simulink model "V3_2_MatlabFn"  (R2017b)
settings: Solver=VariableStepAuto  StartTime=0.0  StopTime=.1  MaxStep=1e-4  RelTol=1e-3
undefined symbols (not defined in the file or in its folder): gain, Ion, L, Lithium, RL
libraries: powerlib x55, simulink x11, nesl_utility x5, fl_lib x4, powerlib_meascontrol x4, elec_lib x3, electricdrivelib x2, simulink_need_slupdate x1, dspswit3 x1
settings Model: Creator=Manu Krishnan  LastModifiedBy=Manu Krishnan

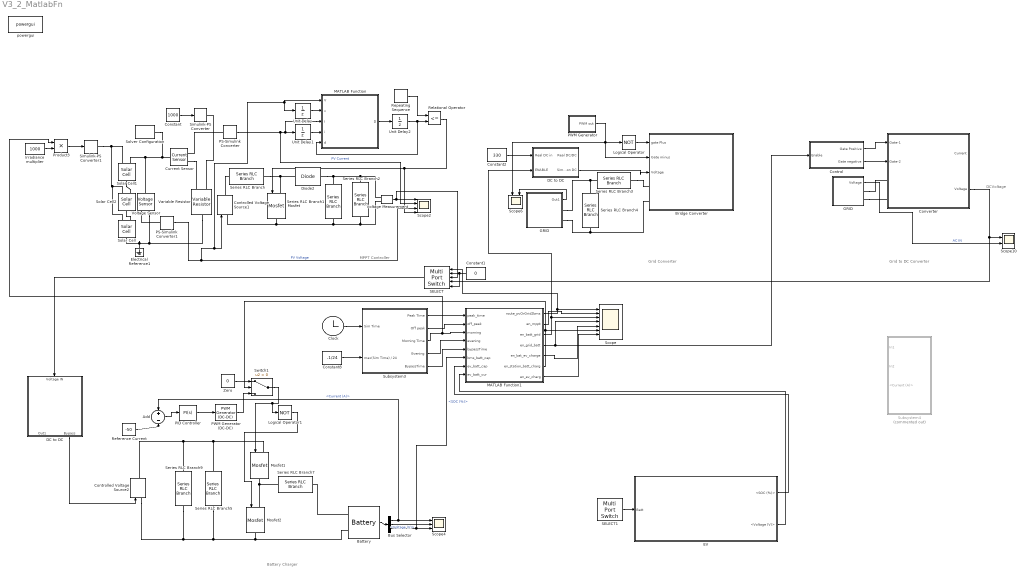
== system V3_2_MatlabFn ==
  note: DCVoltage
  note: Grid Converter
  note: Battery Charger
  note: MPPT Controller
  note: Grid to DC Converter
  Add : Sum  Inputs=+-
  Battery : electricdrivelib/Extra Sources/Battery  BatType=Lithium-Ion  ShowTempParam=off  ThermalPreset=no  ShowAgeParam=on  NomV=300  NomQ=100  SOC=30  Batt_Tr=1  PresetModel=on  MaxQ=100  MinV=225  FullV=349.1961  Dis_rate=43.4783  R=0.03  Normal_OP=90.4348  expZone="[324.1158      4.913043]"  current=[6.5 13 32.5]  Units=Time  Tci=20  NomT=20  T2=-30  MaxQ2=4.8  FullV2=7.1  Normal_OP2=5.655  expZone2="[6.58           1]"  Rca=0.6  ti=2000  Dp=0  Neq0=0  Tsim=1e6  Ta1=25  Qeol=5.4*0.9  Reol=0.013333*1.2  Char_age=[2.3478, 3]  Dis_age=[2.3478, 10]  N1=1500  N2=10500  N3=1000  N4=1400  Ta2=45  N5=950
  Bridge Converter : Subsystem
  Bus Selector : BusSelector  OutputSignals=Current (A),Voltage (V),SOC (%)
  Clock : Clock
  Constant : Constant  Value=1000
  Constant1 : Constant  Value=0
  Constant2 : Constant  Value=330
  Constant8 : Constant  Value=.1/24  VectorParams1D=off
  Control : Subsystem
  Controlled Voltage Source1 : powerlib/Electrical Sources/Controlled Voltage Source  Initialize=on  Source_Type=DC  Amplitude=0  Phase=0  Frequency=0  Measurements=None
  Controlled Voltage Source2 : powerlib/Electrical Sources/Controlled Voltage Source  Initialize=on  Source_Type=DC  Amplitude=0  Phase=0  Frequency=0  Measurements=None
  Converter : Subsystem
  Current Sensor : fl_lib/Electrical/Electrical Sensors/Current Sensor
  DC to DC : Subsystem
  "DC to DC " : Subsystem
  Diode2 : powerlib/Power Electronics/Diode  Ron=0.001  Lon=0  Vf=0.8  IC=0  UseSnubber=0  Rs=500  Cs=250e-9  Measurements=off
  EV : Subsystem
      mask Display: image('C:\Users\Manu Krishnan\Downloads\White-Tesla-Electric-Car-PNG-Free-Download (1).png');
  Electrical Reference1 : fl_lib/Electrical/Electrical Elements/Electrical Reference
  GRID : Subsystem
  "GRID " : Subsystem
  Irradiance multiplier : Constant  Value=1000
  Logical Operator : Logic  Operator=NOT  AllPortsSameDT=off  OutDataTypeStr=boolean
  Logical Operator1 : Logic  Operator=NOT  IconShape=distinctive  AllPortsSameDT=off  OutDataTypeStr=boolean
  MATLAB Function : MATLAB Function  TreatAsAtomicUnit=on
  MATLAB Function1 : MATLAB Function  TreatAsAtomicUnit=on
  Mosfet : powerlib/Power Electronics/Mosfet  Ron=0.1  Lon=0  Rd=0.01  Vfd=0  IC=0  Rs=1e5  Cs=inf  Measurements=off
  Mosfet1 : powerlib/Power Electronics/Mosfet  Ron=0.1  Lon=0  Rd=0.01  Vfd=0  IC=0  Rs=1e5  Cs=inf  Measurements=off
  Mosfet2 : powerlib/Power Electronics/Mosfet  Ron=0.1  Lon=0  Rd=0.01  Vfd=0  IC=0  Rs=1e5  Cs=inf  Measurements=off
  PID Controller : simulink/Continuous/PID Controller  Controller=PI  TimeDomain=Continuous-time  SampleTime=-1  IntegratorMethod=Forward Euler  FilterMethod=Forward Euler  Form=Parallel  UseFilter=on  ControllerParametersSource=internal  P=.005  I=10  D=0  N=100  InitialConditionSource=internal  InitialConditionForIntegrator=0  InitialConditionForFilter=0  ExternalReset=none  LimitOutput=on  UpperSaturationLimit=0.975  LowerSaturationLimit=-inf  LinearizeAsGain=on  AntiWindupMode=none  Kb=1  TrackingMode=off  Kt=1  PParamMin=[]  PParamMax=[]  IParamMin=[]  IParamMax=[]  DParamMin=[]  DParamMax=[]  NParamMin=[]  NParamMax=[]  KbParamMin=[]  KbParamMax=[]  KtParamMin=[]  KtParamMax=[]  POutMin=[]  POutMax=[]  IOutMin=[]  IOutMax=[]  DOutMin=[]  DOutMax=[]  NOutMin=[]  NOutMax=[]  KbOutMin=[]  KbOutMax=[]  KtOutMin=[]  KtOutMax=[]  IntegratorOutMin=[]  IntegratorOutMax=[]  FilterOutMin=[]  FilterOutMax=[]  SumOutMin=[]  SumOutMax=[]  SumI1OutMin=[]  SumI1OutMax=[]  SumI2OutMin=[]  SumI2OutMax=[]  SumI3OutMin=[]  SumI3OutMax=[]  SumDOutMin=[]  SumDOutMax=[]  SaturationOutMin=[]  SaturationOutMax=[]  IntegratorContinuousStateAttributes=''  IntegratorStateMustResolveToSignalObject=off  IntegratorRTWStateStorageClass=Auto  FilterContinuousStateAttributes=''  FilterStateMustResolveToSignalObject=off  FilterRTWStateStorageClass=Auto  DifferentiatorICPrevScaledInput=0  DifferentiatorOutMin=[]  DifferentiatorOutMax=[]  InitialConditionSetting=State (most efficient)  FilterDiffOutCoefMin=[]  FilterDiffOutCoefMax=[]  SumDenOutMin=[]  SumDenOutMax=[]  SumNumOutMin=[]  SumNumOutMax=[]  ReciprocalOutMin=[]  ReciprocalOutMax=[]  DivideOutMin=[]  DivideOutMax=[]  TunerSelectOption=Transfer Function Based (PID Tuner App)
  PS-Simulink Converter : nesl_utility/PS-Simulink Converter  PhysicalDomain=network_engine_domain  SubClassName=ps_output  LeftPortType=input  RightPortType=output  PseudoPeriodic=off  Frequencies=[]  Unit=1  AffineConversion=off
  PS-Simulink Converter1 : nesl_utility/PS-Simulink Converter  PhysicalDomain=network_engine_domain  SubClassName=ps_output  LeftPortType=input  RightPortType=output  PseudoPeriodic=off  Frequencies=[]  Unit=1  AffineConversion=off
  PWM Generator : Subsystem
  PWM Generator (DC-DC) : powerlib_meascontrol/Pulse & Signal Generators/PWM Generator (DC-DC)  Fsw=5000  Ts=5e-6
  Product3 : Product
  Reference Current : Constant  Value=-50
  Relational Operator : RelationalOperator  Operator=<=  OutDataTypeStr=boolean  RndMeth=Simplest
  Repeating Sequence : simulink/Sources/Repeating Sequence  rep_seq_t=[0 0.5 1]/1000  rep_seq_y=[0 1 0]
  SELECT : MultiPortSwitch  DataPortOrder=Zero-based contiguous  DataPortForDefault=Additional data port
  SELECT1 : MultiPortSwitch  DataPortOrder=Zero-based contiguous  DataPortForDefault=Additional data port
  Scope : Scope  NumInputPorts=7
  Scope10 : Scope  NumInputPorts=2
  Scope2 : Scope  NumInputPorts=4
  Scope4 : Scope  NumInputPorts=3
  Scope6 : Scope  NumInputPorts=2
  Series RLC Branch : powerlib/Elements/Series RLC Branch  LConnTagsString=__new0  RConnTagsString=__new0  BranchType=L  Resistance=1  Inductance=1000e-6  SetiL0=off  InitialCurrent=0  Capacitance=1e-6  Setx0=off  InitialVoltage=0  Measurements=None
  Series RLC Branch1 : powerlib/Elements/Series RLC Branch  LConnTagsString=__new0  RConnTagsString=__new0  BranchType=C  Resistance=1  Inductance=100e-3  SetiL0=off  InitialCurrent=0  Capacitance=1000e-6  Setx0=off  InitialVoltage=0  Measurements=None
  Series RLC Branch2 : powerlib/Elements/Series RLC Branch  LConnTagsString=__new0  RConnTagsString=__new0  BranchType=R  Resistance=10  Inductance=100e-3  SetiL0=off  InitialCurrent=0  Capacitance=1e-6  Setx0=off  InitialVoltage=0  Measurements=None
  Series RLC Branch3 : powerlib/Elements/Series RLC Branch  LConnTagsString=__new0  RConnTagsString=__new0  BranchType=L  Resistance=1  Inductance=1e-3  SetiL0=off  InitialCurrent=0  Capacitance=1e-6  Setx0=off  InitialVoltage=0  Measurements=None
  Series RLC Branch4 : powerlib/Elements/Series RLC Branch  LConnTagsString=__new0  RConnTagsString=__new0  BranchType=C  Resistance=1  Inductance=100e-3  SetiL0=off  InitialCurrent=0  Capacitance=100e-6  Setx0=off  InitialVoltage=0  Measurements=None
  Series RLC Branch5 : powerlib/Elements/Series RLC Branch  LConnTagsString=__new0  RConnTagsString=__new0  BranchType=RC  Resistance=0.0001  Inductance=100e-3  SetiL0=off  InitialCurrent=0  Capacitance=1000e-6  Setx0=off  InitialVoltage=0  Measurements=None
  Series RLC Branch7 : powerlib/Elements/Series RLC Branch  LConnTagsString=__new0  RConnTagsString=__new0  BranchType=RL  Resistance=.1  Inductance=5.8e-4  SetiL0=off  InitialCurrent=0  Capacitance=1e-6  Setx0=off  InitialVoltage=0  Measurements=None
  Series RLC Branch9 : powerlib/Elements/Series RLC Branch  LConnTagsString=__new0  RConnTagsString=__new0  BranchType=R  Resistance=100  Inductance=100e-3  SetiL0=off  InitialCurrent=0  Capacitance=1e-6  Setx0=off  InitialVoltage=0  Measurements=None
  Simulink-PS Converter : nesl_utility/Simulink-PS Converter  PhysicalDomain=network_engine_domain  SubClassName=ps_input  LeftPortType=input  RightPortType=output  PseudoPeriodic=off  Frequencies=[]  NoiseDistribution=none  NoiseParameters=[]  Unit=1  AffineConversion=off  FilteringAndDerivatives=provide  SimscapeFilterOrder=1  InputFilterTimeConstant=0.001  UdotUserProvided=0
  Simulink-PS Converter1 : nesl_utility/Simulink-PS Converter  PhysicalDomain=network_engine_domain  SubClassName=ps_input  LeftPortType=input  RightPortType=output  PseudoPeriodic=off  Frequencies=[]  NoiseDistribution=none  NoiseParameters=[]  Unit=1  AffineConversion=off  FilteringAndDerivatives=provide  SimscapeFilterOrder=1  InputFilterTimeConstant=0.001  UdotUserProvided=0
  Solar Cell : elec_lib/Sources/Solar Cell  prm=1  Isc=7.34 A  Voc=3.356 V  Is=1e-6 A  Is2=0 A  Iph=7.34 A  Ir0=1000 W/m^2  ec=1.5  N2=2  Rs=0 Ohm  Rp=inf Ohm  N_series=1  TIPH1=0 1/K  EG=1.11 eV  TXIS1=3  TXIS2=3  TRS1=0  TRP1=0  Tmeas=25 degC  TFIXED=25 degC  thermal_mass=100 J/K  initial_temperature=25 degC
      settings: SourceProductName=Simscape Electronics  SourceProductBaseCode=SN
  Solar Cell1 : elec_lib/Sources/Solar Cell  prm=1  Isc=7.34 A  Voc=3.356 V  Is=1e-6 A  Is2=0 A  Iph=7.34 A  Ir0=1000 W/m^2  ec=1.5  N2=2  Rs=0 Ohm  Rp=inf Ohm  N_series=1  TIPH1=0 1/K  EG=1.11 eV  TXIS1=3  TXIS2=3  TRS1=0  TRP1=0  Tmeas=25 degC  TFIXED=25 degC  thermal_mass=100 J/K  initial_temperature=25 degC
      settings: SourceProductName=Simscape Electronics  SourceProductBaseCode=SN
  Solar Cell2 : elec_lib/Sources/Solar Cell  prm=1  Isc=7.34 A  Voc=3.356 V  Is=1e-6 A  Is2=0 A  Iph=7.34 A  Ir0=1000 W/m^2  ec=1.5  N2=2  Rs=0 Ohm  Rp=inf Ohm  N_series=1  TIPH1=0 1/K  EG=1.11 eV  TXIS1=3  TXIS2=3  TRS1=0  TRP1=0  Tmeas=25 degC  TFIXED=25 degC  thermal_mass=100 J/K  initial_temperature=25 degC
      settings: SourceProductName=Simscape Electronics  SourceProductBaseCode=SN
  Solver Configuration : nesl_utility/Solver Configuration  PhysicalDomain=network_engine_domain  SubClassName=solver  LeftPortType=input  RightPortType=generic  Accelerate=off  Tones=[]  Harmonics=[]  SimulateNoise=off  Profile=off  UseLocalSampling=off  EnableSwitchedLinearOptims=on  FrequencyDomain=off  UseCCode=off  RelTol=0.001  AbsTol=1e-06  MinStep=1e-09  ToWorkspace=off  RevertToSquareIcSolve=off  NumHomotopyIterations=100  PhasorMode=off  PhasorModeNumHarmonics=1  DoDC=off  ResidualTolerance=1e-09  UseLocalSolver=off  LocalSolverChoice=NE_BACKWARD_EULER_ADVANCER  LocalSolverSampleTime=0.001  DoFixedCost=off  MaxNonlinIter=3  MaxModeIter=2  LinearAlgebra=Sparse  DelaysMemoryBudget=1024  AutomaticFiltering=on  FilteringTimeConstant=0.001
  Subsystem3 : Subsystem
  Subsystem4 : Subsystem  Commented=on
  Switch1 : Switch  Criteria=u2 > Threshold
  Unit Delay : UnitDelay  SampleTime=-1
  Unit Delay1 : UnitDelay  SampleTime=-1
  Unit Delay2 : UnitDelay  SampleTime=-1
  Variable Resistor : fl_lib/Electrical/Electrical Elements/Variable Resistor  Rmin=0 Ohm  i_specify=off  i_priority=None  i=0 A  i_nominal_specify=off  i_nominal_unit=A  i_nominal_value=1  v_specify=off  v_priority=None  v=0 V  v_nominal_specify=off  v_nominal_unit=V  v_nominal_value=1
  Voltage Measurement : powerlib/Measurements/Voltage Measurement  PhasorSimulation=off  OutputType=Complex  PSBequivalent=0
  Voltage Sensor : fl_lib/Electrical/Electrical Sensors/Voltage Sensor
  Zero : Constant  Value=0
  powergui : powerlib/powergui  Priority=1  SimulationMode=Continuous  SampleTime=50e-6  frequency=60  Iterations=50  frequencyindice=0  Pbase=100e6  ErrMax=1e-4  UnitsV=kV  UnitsW=MW  buscounter=0  FunctionMessages=off  echomessages=off  EnableUseOfTLC=off  CurrentSourceSwitches=off  DisableSnubberDevices=off  DisableRonSwitches=off  DisableVfSwitches=off  DisplayEquations=off  SolverType=Tustin/Backward Euler (TBE)  Interpol=off  ExternalGateDelay=off  methode=off  Ts=100  x0status=blocks  SPID=on  SwTol=0  HookPort=off  RestoreLinks=warning  ResistiveCurrentMeasurement=off  Frange=[0:2:500]  Ylog=off  Xlog=on  ShowGrid=off  save=off  variable=ZData  structure=0  ZoomFFT=off  StartTime=0.0  cycles=1  DisplayStyle=1  fundamental=60  FreqAxis=off  MaxFrequency=1000  frequencyindicesteady=1  RmsSteady=1  display=off
  wires:
  Constant/1 -> Simulink-PS Converter/1
  PS-Simulink Converter/1 -> Scope2/2, MATLAB Function/3(I), Unit Delay1/1  "PV Current"
  PS-Simulink Converter1/1 -> Unit Delay/1, MATLAB Function/1(V), Controlled Voltage Source1/1, Scope2/3  "PV Voltage"
  Voltage Measurement/1 -> SELECT/3, Scope2/1
  Unit Delay/1 -> MATLAB Function/2(v)
  Unit Delay1/1 -> MATLAB Function/4(i)
  MATLAB Function/1(D) -> Unit Delay2/1
  Unit Delay2/1 -> Relational Operator/2, MATLAB Function/5(d)
  Repeating Sequence/1 -> Relational Operator/1
  Logical Operator/1 -> Bridge Converter/1(gate Plus)
  PWM Generator/1("PWM out ") -> Scope6/1, Bridge Converter/2(Gate minus), Logical Operator/1
  Battery/1 -> Bus Selector/1
  Bus Selector/1 -> Add/1, Scope4/1  "<Current (A)>"
  Bus Selector/3 -> MATLAB Function1/6(bms_batt_cap), Scope4/3  "<SOC (%)>"
  Bus Selector/2 -> Scope4/2  "<Voltage (V)>"
  PID Controller/1 -> PWM Generator (DC-DC)/1
  Logical Operator1/1 -> Mosfet2/1
  Add/1 -> PID Controller/1
  Reference Current/1 -> Add/2
  Control/2(Gate negative) -> Converter/2(Gate-2)
  Control/1(Gate Positive) -> Converter/1(Gate-1)
  "GRID "/1(Voltage) -> Scope10/2  "AC IN"
  Switch1/1 -> Mosfet1/1, Logical Operator1/1
  PWM Generator (DC-DC)/1 -> Switch1/3
  Clock/1 -> Subsystem3/1(Sim Time)
  Constant8/1 -> Subsystem3/2(max(Sim Time) / 24)
  GRID/1(Out1) -> Scope6/2
  Converter/2(Voltage) -> Scope10/1, SELECT/4
  Subsystem3/1(Peak Time) -> MATLAB Function1/1(peak_time)
  Subsystem3/2(Off peak) -> MATLAB Function1/2(off_peak)
  Subsystem3/3(Morning Time) -> MATLAB Function1/3(morning), Product3/1
  Subsystem3/4(Evening) -> MATLAB Function1/4(evening)
  Subsystem3/5(BypassTime) -> MATLAB Function1/5(bypassTime)
  MATLAB Function1/2(en_mppt) -> Scope/2
  MATLAB Function1/3(en_batt_grid) -> Scope/3, DC to DC/2(ENABLE)
  MATLAB Function1/7(en_ev_charg) -> Scope/7
  MATLAB Function1/6(en_station_batt_charg) -> Switch1/2, Scope/6
  Zero/1 -> Switch1/1
  Constant1/1 -> SELECT/5, SELECT/2
  MATLAB Function1/1(route_pvOrGrid2bms) -> SELECT/1, Scope/1
  MATLAB Function1/5(en_bat_ev_charge) -> Scope/5
  Relational Operator/1 -> Scope2/4, Mosfet/1
  Irradiance multiplier/1 -> Product3/2
  Product3/1 -> Simulink-PS Converter1/1
  MATLAB Function1/4(en_grid_batt) -> Scope/4, Control/1(Enable)
  DC to DC/2(Simulation DC) -> Bridge Converter/3(Voltage)
  Constant2/1 -> DC to DC/1(Real DC in)
  "DC to DC "/2(Bypass) -> Controlled Voltage Source2/1
  SELECT/1 -> "DC to DC "/1(Voltage IN)
  EV/1(<SOC (%)>) -> MATLAB Function1/7(ev_batt_cap)
  EV/2(<Voltage (V)>) -> MATLAB Function1/8(ev_batt_cur)
  SELECT1/1 -> EV/1(Batt)
  connections:
  Solar Cell1/RConn1 -- Solar Cell2/LConn2
  Solar Cell2/RConn1 -- Solar Cell/LConn2
  Variable Resistor/RConn1 -- Voltage Sensor/RConn2 -- Electrical Reference1/LConn1 -- Solar Cell/RConn1
  Variable Resistor/LConn1 -- Simulink-PS Converter/RConn1
  Simulink-PS Converter1/RConn1 -- Solar Cell/LConn1 -- Solar Cell2/LConn1 -- Solar Cell1/LConn1
  Solar Cell1/LConn2 -- Voltage Sensor/LConn1 -- Solver Configuration/RConn1 -- Current Sensor/LConn1
  Current Sensor/RConn2 -- Variable Resistor/LConn2
  Current Sensor/RConn1 -- PS-Simulink Converter/LConn1
  Series RLC Branch/RConn1 -- Diode2/LConn1 -- Mosfet/LConn1
  Mosfet/RConn1 -- Voltage Measurement/LConn2 -- Series RLC Branch2/RConn1 -- Series RLC Branch1/RConn1 -- Controlled Voltage Source1/LConn1
  Diode2/RConn1 -- Voltage Measurement/LConn1 -- Series RLC Branch2/LConn1 -- Series RLC Branch1/LConn1
  Controlled Voltage Source1/RConn1 -- Series RLC Branch/LConn1
  Series RLC Branch3/LConn1 -- GRID/RConn1 -- Series RLC Branch4/LConn1
  Series RLC Branch3/RConn1 -- Bridge Converter/LConn1
  Series RLC Branch4/RConn1 -- GRID/RConn2 -- Bridge Converter/LConn2
  Mosfet1/RConn1 -- Mosfet2/LConn1 -- Series RLC Branch7/RConn1
  Battery/LConn1 -- Series RLC Branch7/LConn1
  Battery/LConn2 -- Series RLC Branch5/RConn1 -- Controlled Voltage Source2/LConn1 -- Series RLC Branch9/RConn1 -- Mosfet2/RConn1
  Series RLC Branch5/LConn1 -- Controlled Voltage Source2/RConn1 -- Series RLC Branch9/LConn1 -- Mosfet1/LConn1
  "GRID "/RConn1 -- Converter/LConn1
  "GRID "/RConn2 -- Converter/LConn2
  PS-Simulink Converter1/LConn1 -- Voltage Sensor/RConn1

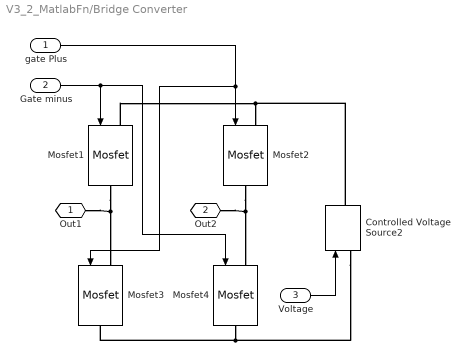
== system V3_2_MatlabFn/Bridge Converter ==
  gate Plus : Inport
  Gate minus : Inport  Port=2
  Voltage : Inport  Port=3
  Controlled Voltage Source2 : powerlib/Electrical Sources/Controlled Voltage Source  Initialize=on  Source_Type=DC  Amplitude=0  Phase=0  Frequency=0  Measurements=None
  Mosfet{1..4} (4 alike) : powerlib/Power Electronics/Mosfet  Ron=0.1  Lon=0  Rd=0.01  Vfd=0  IC=0  Rs=1e5  Cs=inf  Measurements=off
  Out1 : PMIOPort  Port=1  Side=Left
  Out2 : PMIOPort  Port=2  Side=Left
  wires:
  Voltage/1 -> Controlled Voltage Source2/1
  gate Plus/1 -> Mosfet3/1, Mosfet2/1
  Gate minus/1 -> Mosfet4/1, Mosfet1/1
  connections:
  Mosfet1/LConn1 -- Controlled Voltage Source2/RConn1 -- Mosfet2/LConn1
  Mosfet4/RConn1 -- Controlled Voltage Source2/LConn1 -- Mosfet3/RConn1
  Mosfet1/RConn1 -- Out1/RConn1 -- Mosfet3/LConn1
  Mosfet2/RConn1 -- Out2/RConn1 -- Mosfet4/LConn1

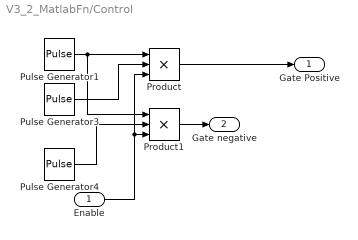
== system V3_2_MatlabFn/Control ==
  Enable : Inport
  Product : Product  Inputs=3
  Product1 : Product  Inputs=3
  Pulse Generator1 : DiscretePulseGenerator  PulseType=Time based  Period=1/25000  PulseWidth=50
  Pulse Generator3 : DiscretePulseGenerator  PulseType=Time based  Period=0.02  PulseWidth=50
  Pulse Generator4 : DiscretePulseGenerator  PulseType=Time based  Period=0.02  PulseWidth=50  PhaseDelay=0.01
  Gate Positive : Outport
  Gate negative : Outport  Port=2
  wires:
  Pulse Generator3/1 -> Product/2
  Pulse Generator1/1 -> Product/1, Product1/1
  Product/1 -> Gate Positive/1
  Product1/1 -> Gate negative/1
  Pulse Generator4/1 -> Product1/2
  Enable/1 -> Product1/3, Product/3

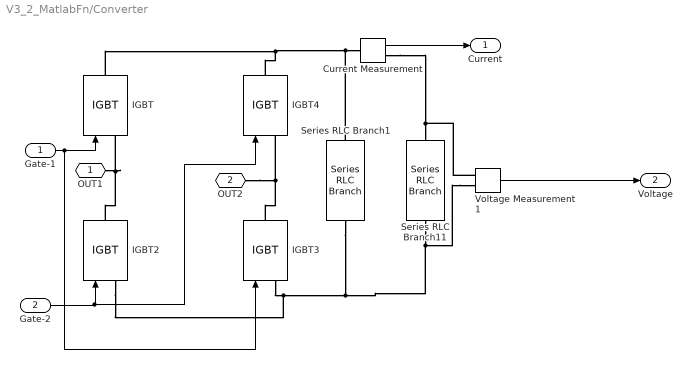
== system V3_2_MatlabFn/Converter ==
  Gate-1 : Inport
  Gate-2 : Inport  Port=2
  Current Measurement : powerlib/Measurements/Current Measurement  PhasorSimulation=off  OutputType=Complex  PSBequivalent=0
  IGBT{,2..4} (4 alike) : powerlib/Power Electronics/IGBT  Ron=0.001  Lon=0  Vf=1  Tf=1e-6  Tt=2e-6  IC=0  Rs=1e5  Cs=inf  Measurements=off
  Series RLC Branch1 : powerlib/Elements/Series RLC Branch  LConnTagsString=__new0  RConnTagsString=__new0  BranchType=C  Resistance=1  Inductance=1e-3  SetiL0=off  InitialCurrent=0  Capacitance=1000e-6  Setx0=off  InitialVoltage=0  Measurements=None
  Series RLC Branch11 : powerlib/Elements/Series RLC Branch  LConnTagsString=__new0  RConnTagsString=__new0  BranchType=R  Resistance=1000  Inductance=1e-3  SetiL0=off  InitialCurrent=0  Capacitance=1e-6  Setx0=off  InitialVoltage=0  Measurements=None
  Voltage Measurement1 : powerlib/Measurements/Voltage Measurement  PhasorSimulation=off  OutputType=Complex  PSBequivalent=0
  OUT1 : PMIOPort  Port=1  Side=Left
  OUT2 : PMIOPort  Port=2  Side=Left
  Current : Outport
  Voltage : Outport  Port=2
  wires:
  Voltage Measurement1/1 -> Voltage/1
  Gate-1/1 -> IGBT3/1, IGBT/1
  Gate-2/1 -> IGBT4/1, IGBT2/1
  Current Measurement/1 -> Current/1
  connections:
  Voltage Measurement1/LConn2 -- Series RLC Branch1/RConn1 -- IGBT2/LConn1 -- IGBT3/LConn1 -- Series RLC Branch11/RConn1
  IGBT4/RConn1 -- IGBT/RConn1 -- Series RLC Branch1/LConn1 -- Current Measurement/LConn1
  Series RLC Branch11/LConn1 -- Current Measurement/RConn1 -- Voltage Measurement1/LConn1
  IGBT/LConn1 -- IGBT2/RConn1 -- OUT1/RConn1
  IGBT4/LConn1 -- IGBT3/RConn1 -- OUT2/RConn1

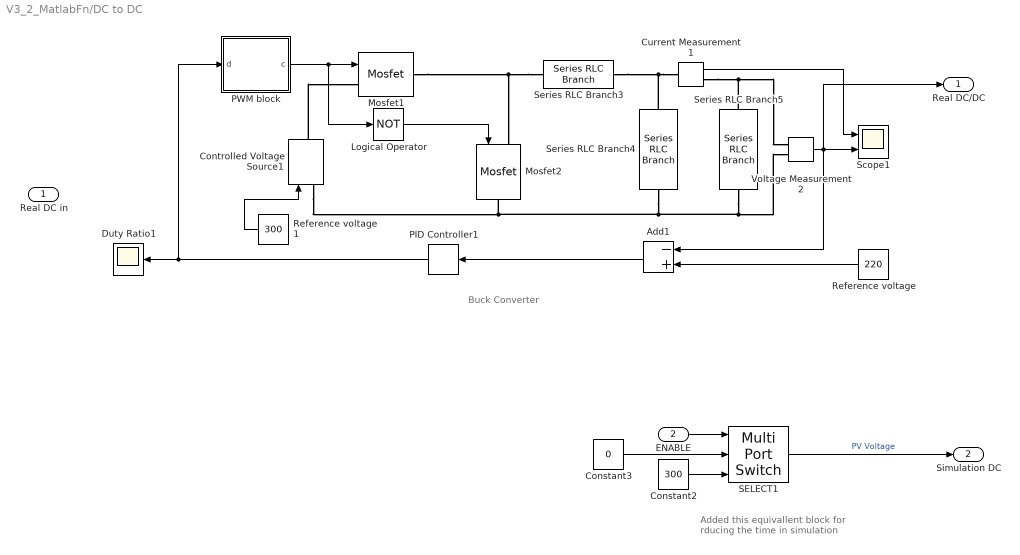
== system V3_2_MatlabFn/DC to DC ==
  note: Added this equivallent block for
      | rducing the time in simulation
  note: Buck Converter
  Real DC in : Inport
  ENABLE : Inport  Port=2
  Add1 : Sum  Inputs=-+
  Constant2 : Constant  Value=300
  Constant3 : Constant  Value=0
  Controlled Voltage Source1 : powerlib/Electrical Sources/Controlled Voltage Source  Initialize=on  Source_Type=DC  Amplitude=200  Phase=0  Frequency=0  Measurements=None
  Current Measurement1 : powerlib/Measurements/Current Measurement  PhasorSimulation=off  OutputType=Complex  PSBequivalent=0
  Duty Ratio1 : Scope
  Logical Operator : Logic  Operator=NOT  AllPortsSameDT=off  OutDataTypeStr=boolean
  Mosfet1 : powerlib/Power Electronics/Mosfet  Ron=0.1  Lon=0  Rd=0.01  Vfd=0  IC=0  Rs=1e5  Cs=inf  Measurements=off
  Mosfet2 : powerlib/Power Electronics/Mosfet  Ron=0.1  Lon=0  Rd=0.01  Vfd=0  IC=0  Rs=1e5  Cs=inf  Measurements=off
  PID Controller1 : simulink_need_slupdate/PID Controller  P=0  I=gain  D=0
      settings: SourceProductName=Simulink
  "PWM block " : Subsystem  mask{fs=100e3}
      mask prompts: fs "Switching fFrequency"
  "Reference voltage   " : Constant  Value=220
  Reference voltage   1 : Constant  Value=300
  SELECT1 : MultiPortSwitch  DataPortOrder=Zero-based contiguous  Inputs=2
  Scope1 : Scope  NumInputPorts=2
  Series RLC Branch3 : powerlib/Elements/Series RLC Branch  LConnTagsString=__new0  RConnTagsString=__new0  BranchType=RL  Resistance=RL  Inductance=L  SetiL0=off  InitialCurrent=0  Capacitance=1e-6  Setx0=off  InitialVoltage=0  Measurements=None
  Series RLC Branch4 : powerlib/Elements/Series RLC Branch  LConnTagsString=__new0  RConnTagsString=__new0  BranchType=R  Resistance=1  Inductance=1e-3  SetiL0=off  InitialCurrent=0  Capacitance=1e-6  Setx0=off  InitialVoltage=0  Measurements=None
  Series RLC Branch5 : powerlib/Elements/Series RLC Branch  LConnTagsString=__new0  RConnTagsString=__new0  BranchType=R  Resistance=1  Inductance=1e-3  SetiL0=off  InitialCurrent=0  Capacitance=1e-6  Setx0=off  InitialVoltage=0  Measurements=None
  Voltage Measurement2 : powerlib/Measurements/Voltage Measurement  PhasorSimulation=off  OutputType=Complex  PSBequivalent=0
  Real DC/DC : Outport
  Simulation DC : Outport  Port=2
  wires:
  PID Controller1/1 -> "PWM block "/1(d), Duty Ratio1/1
  Add1/1 -> PID Controller1/1
  Current Measurement1/1 -> Scope1/1
  "Reference voltage   "/1 -> Add1/2
  "PWM block "/1(c) -> Mosfet1/1, Logical Operator/1
  Logical Operator/1 -> Mosfet2/1
  Voltage Measurement2/1 -> Real DC/DC/1, Scope1/2, Add1/1
  SELECT1/1 -> Simulation DC/1  "PV Voltage"
  Constant3/1 -> SELECT1/2
  ENABLE/1 -> SELECT1/1
  Constant2/1 -> SELECT1/3
  Reference voltage   1/1 -> Controlled Voltage Source1/1
  connections:
  Current Measurement1/LConn1 -- Series RLC Branch4/LConn1 -- Series RLC Branch3/RConn1
  Voltage Measurement2/LConn2 -- Series RLC Branch4/RConn1 -- Controlled Voltage Source1/LConn1 -- Mosfet2/RConn1 -- Series RLC Branch5/RConn1
  Series RLC Branch3/LConn1 -- Mosfet2/LConn1 -- Mosfet1/RConn1
  Current Measurement1/RConn1 -- Series RLC Branch5/LConn1 -- Voltage Measurement2/LConn1
  Controlled Voltage Source1/RConn1 -- Mosfet1/LConn1

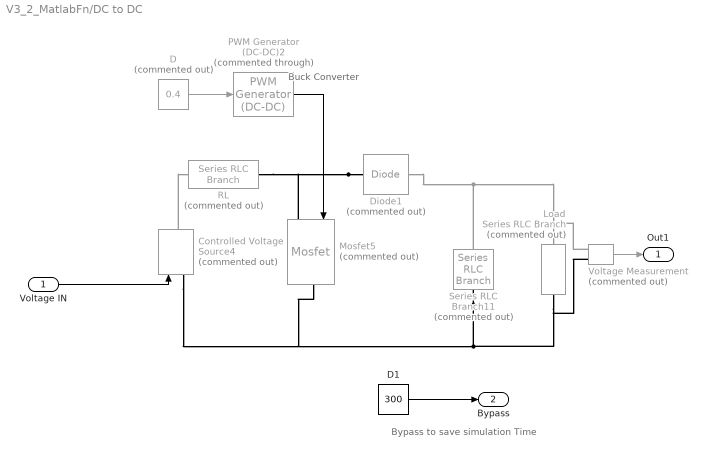
== system V3_2_MatlabFn/DC to DC  ==
  note: Bypass to save simulation Time
  note: Buck Converter
  Voltage IN : Inport
  Controlled Voltage Source4 : powerlib/Electrical Sources/Controlled Voltage Source  Commented=on  Initialize=on  Source_Type=DC  Amplitude=0  Phase=0  Frequency=0  Measurements=None
  D : Constant  Commented=on  Value=0.4
  D1 : Constant  Value=300
  Diode1 : powerlib/Power Electronics/Diode  Commented=on  Ron=1e-3  Lon=0  Vf=0  IC=0  UseSnubber=off  Rs=inf  Cs=inf  Measurements=off
  Load : powerlib/Elements/Series RLC Branch  Commented=on  LConnTagsString=__new0  RConnTagsString=__new0  BranchType=R  Resistance=3  Inductance=200e-6  SetiL0=off  InitialCurrent=0  Capacitance=400e-6  Setx0=off  InitialVoltage=0  Measurements=None
  Mosfet5 : powerlib/Power Electronics/Mosfet  Commented=on  Ron=1e-3  Lon=0  Rd=1e-3  Vfd=0  IC=0  Rs=inf  Cs=inf  Measurements=off
  PWM Generator (DC-DC)2 : powerlib_meascontrol/Pulse & Signal Generators/PWM Generator (DC-DC)  Commented=through  Fsw=20e3  Ts=0
  RL : powerlib/Elements/Series RLC Branch  Commented=on  LConnTagsString=__new0  RConnTagsString=__new0  BranchType=RL  Resistance=1e-3  Inductance=250e-6  SetiL0=off  InitialCurrent=0  Capacitance=1e-6  Setx0=off  InitialVoltage=0  Measurements=None
  Series RLC Branch11 : powerlib/Elements/Series RLC Branch  Commented=on  LConnTagsString=__new0  RConnTagsString=__new0  BranchType=C  Resistance=1e-4  Inductance=200e-6  SetiL0=off  InitialCurrent=0  Capacitance=200e-6  Setx0=off  InitialVoltage=40  Measurements=None
  Voltage Measurement : powerlib/Measurements/Voltage Measurement  Commented=on  PhasorSimulation=off  OutputType=Complex  PSBequivalent=0
  Out1 : Outport
  Bypass : Outport  Port=2
  wires:
  Voltage IN/1 -> Controlled Voltage Source4/1
  D/1 -> PWM Generator (DC-DC)2/1
  PWM Generator (DC-DC)2/1 -> Mosfet5/1
  Voltage Measurement/1 -> Out1/1
  D1/1 -> Bypass/1
  connections:
  Diode1/RConn1 -- Series RLC Branch11/LConn1 -- Voltage Measurement/LConn1 -- Load/LConn1
  Series RLC Branch11/RConn1 -- Voltage Measurement/LConn2 -- Load/RConn1 -- Controlled Voltage Source4/LConn1 -- Mosfet5/RConn1
  Diode1/LConn1 -- RL/RConn1 -- Mosfet5/LConn1
  Controlled Voltage Source4/RConn1 -- RL/LConn1

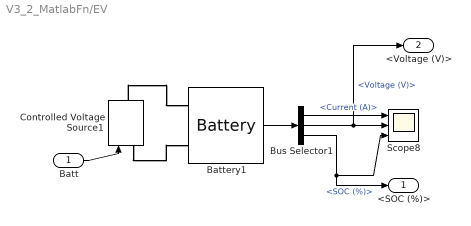
== system V3_2_MatlabFn/EV ==
  Batt : Inport
  Battery1 : electricdrivelib/Extra Sources/Battery  BatType=Lithium-Ion  ShowTempParam=off  ThermalPreset=no  ShowAgeParam=on  NomV=300  NomQ=5.4  SOC=96  Batt_Tr=3  PresetModel=on  MaxQ=5.4  MinV=225  FullV=349.1961  Dis_rate=2.3478  R=0.55556  Normal_OP=4.8835  expZone="[324.1158     0.2653043]"  current=[6.5 13 32.5]  Units=Time  Tci=20  NomT=20  T2=-30  MaxQ2=4.8  FullV2=7.1  Normal_OP2=5.655  expZone2="[6.58           1]"  Rca=0.6  ti=2000  Dp=0  Neq0=0  Tsim=1e6  Ta1=25  Qeol=5.4*0.9  Reol=0.013333*1.2  Char_age=[2.3478, 3]  Dis_age=[2.3478, 10]  N1=1500  N2=10500  N3=1000  N4=1400  Ta2=45  N5=950
  Bus Selector1 : BusSelector  OutputSignals=Current (A),Voltage (V),SOC (%)
  Controlled Voltage Source1 : powerlib/Electrical Sources/Controlled Voltage Source  Initialize=on  Source_Type=DC  Amplitude=0  Phase=0  Frequency=0  Measurements=None
  Scope8 : Scope  NumInputPorts=3
  <SOC (%)> : Outport
  <Voltage (V)> : Outport  Port=2
  wires:
  Bus Selector1/2 -> <Voltage (V)>/1, Scope8/2  "<Voltage (V)>"
  Battery1/1 -> Bus Selector1/1
  Bus Selector1/1 -> Scope8/1  "<Current (A)>"
  Bus Selector1/3 -> <SOC (%)>/1, Scope8/3  "<SOC (%)>"
  Batt/1 -> Controlled Voltage Source1/1
  connections:
  Controlled Voltage Source1/LConn1 -- Battery1/LConn2
  Controlled Voltage Source1/RConn1 -- Battery1/LConn1

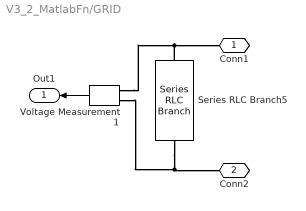
== system V3_2_MatlabFn/GRID ==
  Series RLC Branch5 : powerlib/Elements/Series RLC Branch  LConnTagsString=__new0  RConnTagsString=__new0  BranchType=R  Resistance=1000  Inductance=100e-3  SetiL0=off  InitialCurrent=0  Capacitance=1e-6  Setx0=off  InitialVoltage=0  Measurements=None
  Voltage Measurement1 : powerlib/Measurements/Voltage Measurement  PhasorSimulation=off  OutputType=Complex  PSBequivalent=0
  Conn1 : PMIOPort  Port=1  Side=Right
  Conn2 : PMIOPort  Port=2  Side=Right
  Out1 : Outport
  wires:
  Voltage Measurement1/1 -> Out1/1
  connections:
  Series RLC Branch5/LConn1 -- Conn1/RConn1 -- Voltage Measurement1/LConn2
  Voltage Measurement1/LConn1 -- Conn2/RConn1 -- Series RLC Branch5/RConn1

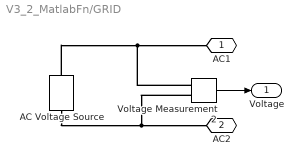
== system V3_2_MatlabFn/GRID  ==
  AC Voltage Source : powerlib/Electrical Sources/AC Voltage Source  Amplitude=230  Phase=0  Frequency=50  SampleTime=0  Measurements=None  BusType=swing  Pref=10e3  Qref=0  Qmin=-inf  Qmax=+inf
  Voltage Measurement2 : powerlib/Measurements/Voltage Measurement  PhasorSimulation=off  OutputType=Complex  PSBequivalent=0
  AC1 : PMIOPort  Port=1  Side=Right
  AC2 : PMIOPort  Port=2  Side=Right
  Voltage : Outport
  wires:
  Voltage Measurement2/1 -> Voltage/1
  connections:
  AC Voltage Source/LConn1 -- AC2/RConn1 -- Voltage Measurement2/LConn2
  AC Voltage Source/RConn1 -- Voltage Measurement2/LConn1 -- AC1/RConn1

== system V3_2_MatlabFn/PWM Generator ==
  Relational Operator1 : RelationalOperator  OutDataTypeStr=boolean  RndMeth=Simplest
  Sawtooth Generator : powerlib_meascontrol/Pulse & Signal Generators/Sawtooth Generator  Freq=10e3  Phase=180  Ts=0
      settings: SourceProductName=Simscape Power Systems
  Sine Wave : Sin  Frequency=314.18  SampleTime=0
  "PWM out " : Outport
  wires:
  Sine Wave/1 -> Relational Operator1/1
  Sawtooth Generator/1 -> Relational Operator1/2
  Relational Operator1/1 -> "PWM out "/1

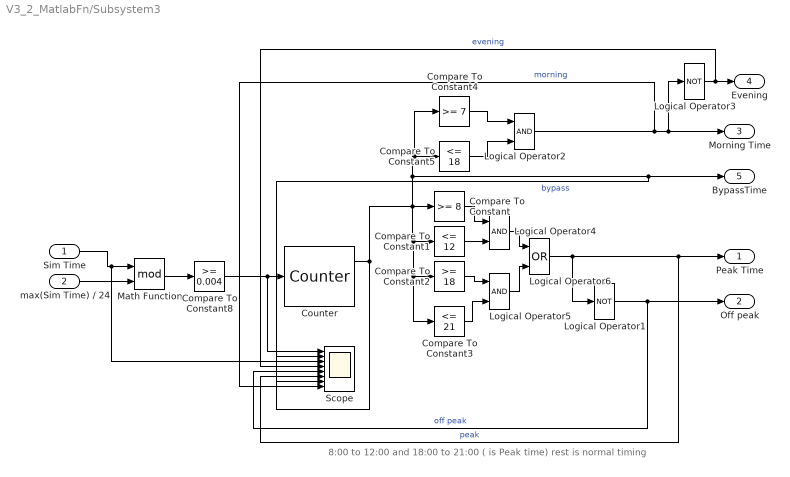
== system V3_2_MatlabFn/Subsystem3 ==
  note: 8:00 to 12:00 and 18:00 to 21:00 ( is Peak time)
      | rest is normal timing
  Sim Time : Inport
  max(Sim Time) / 24 : Inport  Port=2
  Compare To Constant : simulink/Logic and Bit Operations/Compare To Constant  relop=>=  const=8  OutDataTypeStr=boolean  ZeroCross=off
  Compare To Constant1 : simulink/Logic and Bit Operations/Compare To Constant  relop=<=  const=12  OutDataTypeStr=boolean  ZeroCross=off
  Compare To Constant2 : simulink/Logic and Bit Operations/Compare To Constant  relop=>=  const=18  OutDataTypeStr=boolean  ZeroCross=off
  Compare To Constant3 : simulink/Logic and Bit Operations/Compare To Constant  relop=<=  const=21  OutDataTypeStr=boolean  ZeroCross=off
  Compare To Constant4 : simulink/Logic and Bit Operations/Compare To Constant  relop=>=  const=7  OutDataTypeStr=boolean  ZeroCross=off
  Compare To Constant5 : simulink/Logic and Bit Operations/Compare To Constant  relop=<=  const=18  OutDataTypeStr=boolean  ZeroCross=off
  Compare To Constant8 : simulink/Logic and Bit Operations/Compare To Constant  relop=>=  const=0.004  OutDataTypeStr=boolean  ZeroCross=off
  Counter : dspswit3/Counter  Direction=Up  CountEvent=Falling edge  CounterSize=User defined  MaxCount=24  InitialCount=0  Output=Count and Hit  HitValue=24  ResetInput=off  SamplesPerFrame=1  Ts=1  CntDtype=int8  HitDtype=Logical
  Logical Operator1 : Logic  Operator=NOT  AllPortsSameDT=off  OutDataTypeStr=boolean
  Logical Operator2 : Logic  AllPortsSameDT=off  OutDataTypeStr=boolean
  Logical Operator3 : Logic  Operator=NOT  AllPortsSameDT=off  OutDataTypeStr=boolean
  Logical Operator4 : Logic  AllPortsSameDT=off  OutDataTypeStr=boolean
  Logical Operator5 : Logic  AllPortsSameDT=off  OutDataTypeStr=boolean
  Logical Operator6 : Logic  Operator=OR  AllPortsSameDT=off  OutDataTypeStr=boolean
  Math Function : Math  Operator=mod  SaturateOnIntegerOverflow=on
  Scope : Scope  NumInputPorts=8
  Peak Time : Outport
  Off peak : Outport  Port=2
  Morning Time : Outport  Port=3
  Evening : Outport  Port=4
  BypassTime : Outport  Port=5
  wires:
  Sim Time/1 -> Scope/3, Math Function/1
  Logical Operator5/1 -> Logical Operator6/2
  Logical Operator4/1 -> Logical Operator6/1
  Compare To Constant1/1 -> Logical Operator4/2
  Compare To Constant3/1 -> Logical Operator5/2
  Compare To Constant/1 -> Logical Operator4/1
  Logical Operator6/1 -> Logical Operator1/1, Scope/6, Peak Time/1  "peak"
  Math Function/1 -> Compare To Constant8/1
  Logical Operator1/1 -> Scope/5, Off peak/1  "off peak"
  Compare To Constant4/1 -> Logical Operator2/1
  Compare To Constant5/1 -> Logical Operator2/2
  Logical Operator2/1 -> Scope/8, Logical Operator3/1, Morning Time/1  "morning"
  Compare To Constant2/1 -> Logical Operator5/1
  Logical Operator3/1 -> Scope/4, Evening/1  "evening"
  max(Sim Time) / 24/1 -> Math Function/2
  Compare To Constant8/1 -> Scope/1, Counter/1
  Counter/1 -> Scope/2, Scope/7, BypassTime/1, Compare To Constant5/1, Compare To Constant4/1, Compare To Constant3/1, Compare To Constant2/1, Compare To Constant1/1, Compare To Constant/1  "bypass"

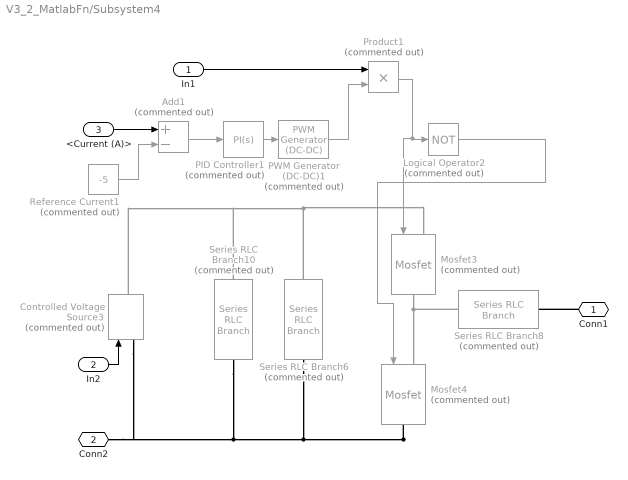
== system V3_2_MatlabFn/Subsystem4 ==
  In1 : Inport
  In2 : Inport  Port=2
  <Current (A)> : Inport  Port=3
  Add1 : Sum  Commented=on  Inputs=+-
  Controlled Voltage Source3 : powerlib/Electrical Sources/Controlled Voltage Source  Commented=on  Initialize=on  Source_Type=DC  Amplitude=0  Phase=0  Frequency=0  Measurements=None
  Logical Operator2 : Logic  Commented=on  Operator=NOT  AllPortsSameDT=off  OutDataTypeStr=boolean
  Mosfet3 : powerlib/Power Electronics/Mosfet  Commented=on  Ron=0.1  Lon=0  Rd=0.01  Vfd=0  IC=0  Rs=1e5  Cs=inf  Measurements=off
  Mosfet4 : powerlib/Power Electronics/Mosfet  Commented=on  Ron=0.1  Lon=0  Rd=0.01  Vfd=0  IC=0  Rs=1e5  Cs=inf  Measurements=off
  PID Controller1 : simulink/Continuous/PID Controller  Commented=on  Controller=PI  TimeDomain=Continuous-time  SampleTime=-1  IntegratorMethod=Forward Euler  FilterMethod=Forward Euler  Form=Parallel  UseFilter=on  ControllerParametersSource=internal  P=.005  I=10  D=0.05  N=100  InitialConditionSource=internal  InitialConditionForIntegrator=0  InitialConditionForFilter=0  ExternalReset=none  LimitOutput=on  UpperSaturationLimit=0.975  LowerSaturationLimit=-inf  LinearizeAsGain=on  AntiWindupMode=none  Kb=1  TrackingMode=off  Kt=1  PParamMin=[]  PParamMax=[]  IParamMin=[]  IParamMax=[]  DParamMin=[]  DParamMax=[]  NParamMin=[]  NParamMax=[]  KbParamMin=[]  KbParamMax=[]  KtParamMin=[]  KtParamMax=[]  POutMin=[]  POutMax=[]  IOutMin=[]  IOutMax=[]  DOutMin=[]  DOutMax=[]  NOutMin=[]  NOutMax=[]  KbOutMin=[]  KbOutMax=[]  KtOutMin=[]  KtOutMax=[]  IntegratorOutMin=[]  IntegratorOutMax=[]  FilterOutMin=[]  FilterOutMax=[]  SumOutMin=[]  SumOutMax=[]  SumI1OutMin=[]  SumI1OutMax=[]  SumI2OutMin=[]  SumI2OutMax=[]  SumI3OutMin=[]  SumI3OutMax=[]  SumDOutMin=[]  SumDOutMax=[]  SaturationOutMin=[]  SaturationOutMax=[]  IntegratorContinuousStateAttributes=''  IntegratorStateMustResolveToSignalObject=off  IntegratorRTWStateStorageClass=Auto  FilterContinuousStateAttributes=''  FilterStateMustResolveToSignalObject=off  FilterRTWStateStorageClass=Auto  DifferentiatorICPrevScaledInput=0  DifferentiatorOutMin=[]  DifferentiatorOutMax=[]  InitialConditionSetting=State (most efficient)  FilterDiffOutCoefMin=[]  FilterDiffOutCoefMax=[]  SumDenOutMin=[]  SumDenOutMax=[]  SumNumOutMin=[]  SumNumOutMax=[]  ReciprocalOutMin=[]  ReciprocalOutMax=[]  DivideOutMin=[]  DivideOutMax=[]  TunerSelectOption=Transfer Function Based (PID Tuner App)
  PWM Generator (DC-DC)1 : powerlib_meascontrol/Pulse & Signal Generators/PWM Generator (DC-DC)  Commented=on  Fsw=5000  Ts=5e-6
  Product1 : Product  Commented=on
  Reference Current1 : Constant  Commented=on  Value=-5
  Series RLC Branch10 : powerlib/Elements/Series RLC Branch  Commented=on  LConnTagsString=__new0  RConnTagsString=__new0  BranchType=R  Resistance=100  Inductance=100e-3  SetiL0=off  InitialCurrent=0  Capacitance=1e-6  Setx0=off  InitialVoltage=0  Measurements=None
  Series RLC Branch6 : powerlib/Elements/Series RLC Branch  Commented=on  LConnTagsString=__new0  RConnTagsString=__new0  BranchType=RC  Resistance=0.0001  Inductance=100e-3  SetiL0=off  InitialCurrent=0  Capacitance=1000e-6  Setx0=off  InitialVoltage=0  Measurements=None
  Series RLC Branch8 : powerlib/Elements/Series RLC Branch  Commented=on  LConnTagsString=__new0  RConnTagsString=__new0  BranchType=RL  Resistance=.1  Inductance=5.8e-4  SetiL0=off  InitialCurrent=0  Capacitance=1e-6  Setx0=off  InitialVoltage=0  Measurements=None
  Conn1 : PMIOPort  Port=1  Side=Left
  Conn2 : PMIOPort  Port=2  Side=Right
  wires:
  <Current (A)>/1 -> Add1/1
  In1/1 -> Product1/1
  PID Controller1/1 -> PWM Generator (DC-DC)1/1
  Logical Operator2/1 -> Mosfet4/1
  PWM Generator (DC-DC)1/1 -> Product1/2
  Product1/1 -> Mosfet3/1, Logical Operator2/1
  Add1/1 -> PID Controller1/1
  Reference Current1/1 -> Add1/2
  In2/1 -> Controlled Voltage Source3/1
  connections:
  Conn1/RConn1 -- Series RLC Branch8/LConn1
  Mosfet3/RConn1 -- Mosfet4/LConn1 -- Series RLC Branch8/RConn1
  Series RLC Branch6/LConn1 -- Controlled Voltage Source3/RConn1 -- Series RLC Branch10/LConn1 -- Mosfet3/LConn1
  Mosfet4/RConn1 -- Series RLC Branch6/RConn1 -- Series RLC Branch10/RConn1 -- Controlled Voltage Source3/LConn1 -- Conn2/RConn1

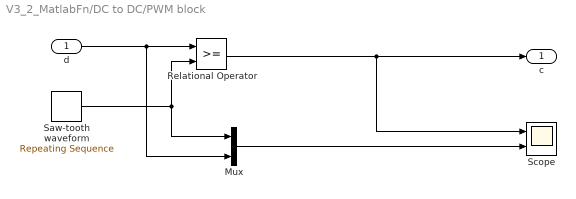
== system V3_2_MatlabFn/DC to DC/PWM block  ==
  d : Inport
  Mux : Mux  Inputs=2
  Relational Operator : RelationalOperator  OutDataTypeStr=boolean  RndMeth=Nearest
  Saw-tooth waveform : simulink/Sources/Repeating Sequence  rep_seq_t=[0 1/fs]  rep_seq_y=[0 1]
  Scope : Scope  NumInputPorts=2
  c : Outport
  wires:
  Mux/1 -> Scope/2
  Relational Operator/1 -> Scope/1, c/1
  Saw-tooth waveform/1 -> Relational Operator/2, Mux/1
  d/1 -> Relational Operator/1, Mux/2

== matlab function V3_2_MatlabFn/MATLAB Function1 ==
  data: route_pvOrGrid2bms output; en_mppt output; en_batt_grid output; en_grid_batt output; en_bat_ev_charge output; en_station_batt_charg output; en_ev_charg output; peak_time input; off_peak input; morning input; evening input; bypassTime input; bms_batt_cap input; ev_batt_cap input; ev_batt_cur input
function [route_pvOrGrid2bms, en_mppt,en_batt_grid, en_grid_batt, en_bat_ev_charge, en_station_batt_charg,en_ev_charg]= Automate(peak_time,off_peak,morning,evening,bypassTime,bms_batt_cap,ev_batt_cap,ev_batt_cur)
from_grid = 2;
from_solar =1;
if(ev_batt_cur < 1)
    carPresent = 0;
else
    carPresent =1;
end

% MODE 1 
% PV to battery
%---------------------------------------------------------------------------------------
%Time	        |Speicific Time	|EV 	             |BatteryBank Capacity	|EV battery
%---------------------------------------------------------------------------------------
%Morning 	    |Off peak	    |Not present         |<80%	                |>90%
%---------------------------------------------------------------------------------------
if  (off_peak &&   carPresent==0 && bms_batt_cap < 80 && ev_batt_cap > 90)
    en_station_batt_charg =1;
    en_mppt =1;
    route_pvOrGrid2bms =from_solar;
    en_batt_grid =0;
    en_grid_batt =0;
    en_ev_charg =0;
    en_bat_ev_charge =0;
%####################################################################################### 
% MODE 2
% PV to Electric Vehicle 
%---------------------------------------------------------------------------------------
%Time	        |Speicific Time	|EV 	             |BatteryBank Capacity	|EV battery
%---------------------------------------------------------------------------------------
%Morning 	    |Off peak	    |Present             |NA	                |<90%
% 
%---------------------------------------------------------------------------------------
elseif (off_peak && morning &&  carPresent==1 && ev_batt_cap < 90)
    en_station_batt_charg =1;
    en_mppt =1;
    route_pvOrGrid2bms =from_solar;
    en_batt_grid =0;
    en_grid_batt =0;
    en_ev_charg =0;
    en_bat_ev_charge =0;
%#######################################################################################    
% MODE 3
% Battery Bank to EV 
%---------------------------------------------------------------------------------------
%Time	        |Speicific Time	|EV 	             |BatteryBank Capacity	|EV battery
%---------------------------------------------------------------------------------------
%Evening	    |18:00 to 21:00	|Present	         | >30%                 |	<90%
%---------------------------------------------------------------------------------------
elseif (peak_time && evening &&  carPresent==1 && bms_batt_cap >30 && ev_batt_cap < 90)
    en_station_batt_charg =1;
    en_mppt =1;
    route_pvOrGrid2bms =from_grid;
    en_batt_grid =0;
    en_grid_batt =0;
    en_ev_charg =1;
    en_bat_ev_charge =1;   
%#######################################################################################  
% MODE 4
% AC grid to EV
%---------------------------------------------------------------------------------------
%Time	        |Speicific Time	|EV 	             |BatteryBank Capacity	|EV battery
%---------------------------------------------------------------------------------------
%Morning 	    |Off peak	    |Not present         |<80%	                |>90%
%---------------------------------------------------------------------------------------
elseif (off_peak && morning &&   carPresent==0 && bms_batt_cap <80 && ev_batt_cap < 90)
    en_station_batt_charg =1;
    en_mppt =1;
    route_pvOrGrid2bms =from_grid;
    en_batt_grid =0;
    en_grid_batt =0;
    en_ev_charg =1;
    en_bat_ev_charge =0;
%#######################################################################################  
% MODE 5
%PV to AC grid 
%---------------------------------------------------------------------------------------
%Time	        |Speicific Time	|EV 	             |BatteryBank Capacity	|EV battery
%---------------------------------------------------------------------------------------
%Morning 	    |NA	            |Not present         |<80%	                |>90%
%---------------------------------------------------------------------------------------
elseif (morning &&  bms_batt_cap >90 && carPresent==0  && ev_batt_cap > 90)
    en_station_batt_charg =1;
    en_mppt =1;
    route_pvOrGrid2bms =from_grid;
    en_batt_grid =0;
    en_grid_batt =0;
    en_ev_charg =0;
    en_bat_ev_charge =0;
else
    en_station_batt_charg =0;
    en_mppt =0;
    route_pvOrGrid2bms =from_grid;
    en_batt_grid =0;
    en_grid_batt =0;
    en_ev_charg =0;
    en_bat_ev_charge =0;

end

== matlab function V3_2_MatlabFn/MATLAB Function ==
  data: V input; D output; v input; I input; i input; d input
function D = MPPT(V,v,I,i,d)

d = 0.58;

dv = V-v;
di = I-i;
if(dv==0)
    if(di==0)
        D=d
    else
        if(di>0)
            D=d+0.05;
        else
            D=d-0.05;
        end
    end
end
if(di/dv == (I/V))
    D=d;
else
    if(di/dv >(I/V))
        D=d+0.05;
    else
        D=d-0.05;
    end
end
